simulink model "PLL_Simulering"  (R2020a)
settings: Solver=VariableStepAuto  StartTime=0  StopTime=0.5  RelTol=1e-3
InitFcn:
  | clear all;
libraries: powerlib x48, eePowerMeasurement x1, powerlib_meascontrol x1
(part 2 of 3)

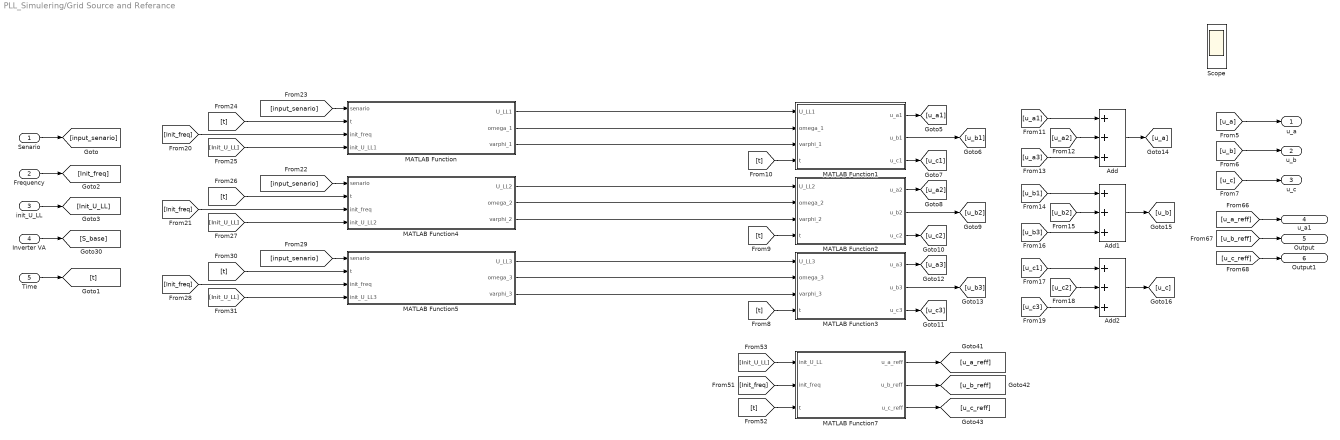
== system PLL_Simulering/Grid Source and Referance ==
  Senario : Inport
  Frequency : Inport  Port=2
  init_U_LL : Inport  Port=3
  Inverter VA : Inport  Port=4
  Time : Inport  Port=5
  Add : Sum  Inputs=+++
  Add1 : Sum  Inputs=+++
  Add2 : Sum  Inputs=+++
  MATLAB Function : MATLAB Function  TreatAsAtomicUnit=on
  MATLAB Function1 : MATLAB Function  TreatAsAtomicUnit=on
  MATLAB Function2 : MATLAB Function  TreatAsAtomicUnit=on
  MATLAB Function3 : MATLAB Function  TreatAsAtomicUnit=on
  MATLAB Function4 : MATLAB Function  TreatAsAtomicUnit=on
  MATLAB Function5 : MATLAB Function  TreatAsAtomicUnit=on
  MATLAB Function7 : MATLAB Function  TreatAsAtomicUnit=on
  Scope : Scope
  u_a : Outport
  u_b : Outport  Port=2
  u_c : Outport  Port=3
  u_a1 : Outport  Port=4
  Output : Outport  Port=5
  Output1 : Outport  Port=6
  wires:
  Senario/1 -> [input_senario]
  [u_a] -> u_a/1
  [u_c] -> u_c/1
  [u_b] -> u_b/1
  Frequency/1 -> [Init_freq]
  [t] -> MATLAB Function3/4(t)
  [t] -> MATLAB Function2/4(t)
  [t] -> MATLAB Function1/4(t)
  MATLAB Function/1(U_LL1) -> MATLAB Function1/1(U_LL1)
  MATLAB Function/2(omega_1) -> MATLAB Function1/2(omega_1)
  MATLAB Function/3(varphi_1) -> MATLAB Function1/3(varphi_1)
  init_U_LL/1 -> [Init_U_LL]
  MATLAB Function4/1(U_LL2) -> MATLAB Function2/1(U_LL2)
  MATLAB Function4/2(omega_2) -> MATLAB Function2/2(omega_2)
  MATLAB Function4/3(varphi_2) -> MATLAB Function2/3(varphi_2)
  MATLAB Function1/1(u_a1) -> [u_a1]
  MATLAB Function1/2(u_b1) -> [u_b1]
  MATLAB Function1/3(u_c1) -> [u_c1]
  MATLAB Function2/3(u_c2) -> [u_c2]
  MATLAB Function2/2(u_b2) -> [u_b2]
  MATLAB Function2/1(u_a2) -> [u_a2]
  MATLAB Function3/2(u_b3) -> [u_b3]
  MATLAB Function3/1(u_a3) -> [u_a3]
  MATLAB Function3/3(u_c3) -> [u_c3]
  [u_a1] -> Add/1
  [u_a2] -> Add/2
  [u_a3] -> Add/3
  [u_b2] -> Add1/2
  [u_b3] -> Add1/3
  [u_b1] -> Add1/1
  [u_c3] -> Add2/3
  [u_c1] -> Add2/1
  [u_c2] -> Add2/2
  Add/1 -> [u_a]
  Add1/1 -> [u_b]
  Add2/1 -> [u_c]
  [input_senario] -> MATLAB Function/1(senario)
  [t] -> MATLAB Function/2(t)
  [Init_U_LL] -> MATLAB Function/4(init_U_LL1)
  [Init_freq] -> MATLAB Function/3(init_freq)
  [Init_freq] -> MATLAB Function4/3(init_freq)
  [Init_U_LL] -> MATLAB Function4/4(init_U_LL2)
  [input_senario] -> MATLAB Function4/1(senario)
  [t] -> MATLAB Function4/2(t)
  [Init_U_LL] -> MATLAB Function5/4(init_U_LL3)
  [input_senario] -> MATLAB Function5/1(senario)
  [t] -> MATLAB Function5/2(t)
  [Init_freq] -> MATLAB Function5/3(init_freq)
  MATLAB Function5/3(varphi_3) -> MATLAB Function3/3(varphi_3)
  MATLAB Function5/2(omega_3) -> MATLAB Function3/2(omega_3)
  MATLAB Function5/1(U_LL3) -> MATLAB Function3/1(U_LL3)
  [t] -> MATLAB Function7/3(t)
  [Init_U_LL] -> MATLAB Function7/1(init_U_LL)
  [Init_freq] -> MATLAB Function7/2(init_freq)
  Inverter VA/1 -> [S_base]
  [u_a_reff] -> u_a1/1
  MATLAB Function7/1(u_a_reff) -> [u_a_reff]
  MATLAB Function7/2(u_b_reff) -> [u_b_reff]
  MATLAB Function7/3(u_c_reff) -> [u_c_reff]
  [u_b_reff] -> Output/1
  [u_c_reff] -> Output1/1
  Time/1 -> [t]

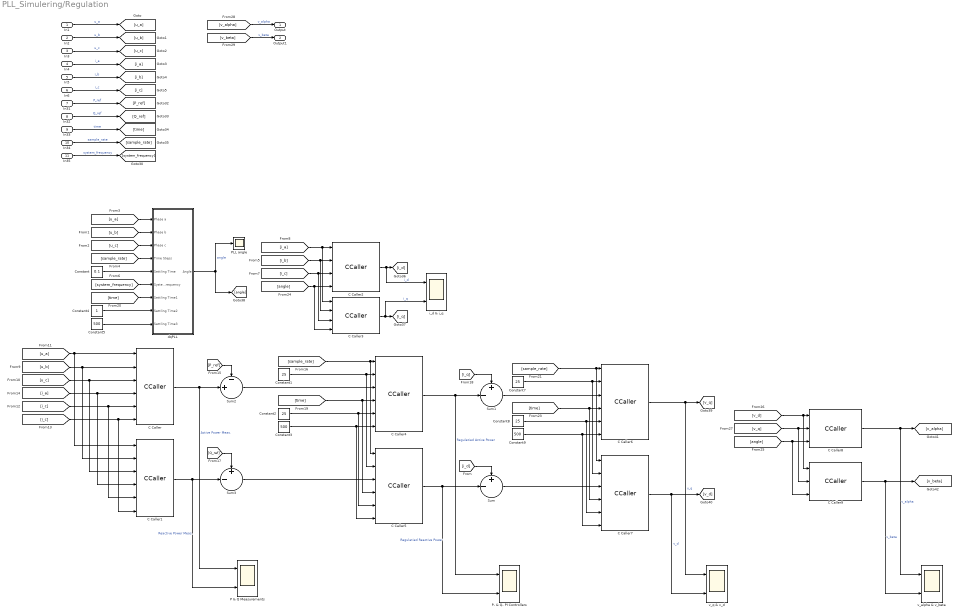
== system PLL_Simulering/Regulation ==
  In1 : Inport
  In2 : Inport  Port=2
  In3 : Inport  Port=3
  In4 : Inport  Port=4
  In5 : Inport  Port=5
  In6 : Inport  Port=6
  In31 : Inport  Port=7
  In32 : Inport  Port=8
  In33 : Inport  Port=9
  In34 : Inport  Port=10
  In35 : Inport  Port=11
  C Caller : CCaller  FunctionName=measure_P  PortSpecificationStruct="%)30     .    V L   8    (     @         %    \"     <    !     0         %  0 \"0    $    _    07)G3F%M90  4&]R=$YA;64 4V-O<&4     26YD97@     5'EP90      4VEZ90      27-';&]B86P   X    P    !@    @    $          4    (     0    ,    !         !   P!O=70 #@   #     &    \"     0         !0    @    !     P    $         $  # &]U=  .    .     8    (    !          %    \"     $    &     0         0   ...(+3703 chars)"
  C Caller1 : CCaller  FunctionName=measure_Q  PortSpecificationStruct="%)30     .    V L   8    (     @         %    \"     <    !     0         %  0 \"0    $    _    07)G3F%M90  4&]R=$YA;64 4V-O<&4     26YD97@     5'EP90      4VEZ90      27-';&]B86P   X    P    !@    @    $          4    (     0    ,    !         !   P!O=70 #@   #     &    \"     0         !0    @    !     P    $         $  # &]U=  .    .     8    (    !          %    \"     $    &     0         0   ...(+3703 chars)"
  C Caller2 : CCaller  FunctionName=Clarke_Park_d  PortSpecificationStruct="%)30     .    J @   8    (     @         %    \"     4    !     0         %  0 \"0    $    _    07)G3F%M90  4&]R=$YA;64 4V-O<&4     26YD97@     5'EP90      4VEZ90      27-';&]B86P   X    P    !@    @    $          4    (     0    ,    !         !   P!O=70 #@   #     &    \"     0         !0    @    !     P    $         $  # &]U=  .    .     8    (    !          %    \"     $    &     0         0   ...(+2601 chars)"
  C Caller3 : CCaller  FunctionName=Clarke_Park_q  PortSpecificationStruct="%)30     .    J @   8    (     @         %    \"     4    !     0         %  0 \"0    $    _    07)G3F%M90  4&]R=$YA;64 4V-O<&4     26YD97@     5'EP90      4VEZ90      27-';&]B86P   X    P    !@    @    $          4    (     0    ,    !         !   P!O=70 #@   #     &    \"     0         !0    @    !     P    $         $  # &]U=  .    .     8    (    !          %    \"     $    &     0         0   ...(+2601 chars)"
  C Caller4 : CCaller  FunctionName=PID_Type_1_1  PortSpecificationStruct="%)30     .    * P   8    (     @         %    \"     <    !     0         %  0 \"0    $    _    07)G3F%M90  4&]R=$YA;64 4V-O<&4     26YD97@     5'EP90      4VEZ90      27-';&]B86P   X    P    !@    @    $          4    (     0    ,    !         !   P!O=70 #@   #     &    \"     0         !0    @    !     P    $         $  # &]U=  .    .     8    (    !          %    \"     $    &     0         0   ...(+3810 chars)"
  C Caller5 : CCaller  FunctionName=PID_Type_1_2  PortSpecificationStruct="%)30     .    * P   8    (     @         %    \"     <    !     0         %  0 \"0    $    _    07)G3F%M90  4&]R=$YA;64 4V-O<&4     26YD97@     5'EP90      4VEZ90      27-';&]B86P   X    P    !@    @    $          4    (     0    ,    !         !   P!O=70 #@   #     &    \"     0         !0    @    !     P    $         $  # &]U=  .    .     8    (    !          %    \"     $    &     0         0   ...(+3810 chars)"
  C Caller6 : CCaller  FunctionName=PID_Type_1_3  PortSpecificationStruct="%)30     .    * P   8    (     @         %    \"     <    !     0         %  0 \"0    $    _    07)G3F%M90  4&]R=$YA;64 4V-O<&4     26YD97@     5'EP90      4VEZ90      27-';&]B86P   X    P    !@    @    $          4    (     0    ,    !         !   P!O=70 #@   #     &    \"     0         !0    @    !     P    $         $  # &]U=  .    .     8    (    !          %    \"     $    &     0         0   ...(+3810 chars)"
  C Caller7 : CCaller  FunctionName=PID_Type_1_4  PortSpecificationStruct="%)30     .    * P   8    (     @         %    \"     <    !     0         %  0 \"0    $    _    07)G3F%M90  4&]R=$YA;64 4V-O<&4     26YD97@     5'EP90      4VEZ90      27-';&]B86P   X    P    !@    @    $          4    (     0    ,    !         !   P!O=70 #@   #     &    \"     0         !0    @    !     P    $         $  # &]U=  .    .     8    (    !          %    \"     $    &     0         0   ...(+3810 chars)"
  C Caller8 : CCaller  FunctionName=Park_inv_alpha  PortSpecificationStruct="%)30     .    \" <   8    (     @         %    \"     0    !     0         %  0 \"0    $    _    07)G3F%M90  4&]R=$YA;64 4V-O<&4     26YD97@     5'EP90      4VEZ90      27-';&]B86P   X    P    !@    @    $          4    (     0    ,    !         !   P!O=70 #@   #     &    \"     0         !0    @    !     P    $         $  # &]U=  .    .     8    (    !          %    \"     $    &     0         0  ...(+2044 chars)"
  C Caller9 : CCaller  FunctionName=Park_inv_beta  PortSpecificationStruct="%)30     .    \" <   8    (     @         %    \"     0    !     0         %  0 \"0    $    _    07)G3F%M90  4&]R=$YA;64 4V-O<&4     26YD97@     5'EP90      4VEZ90      27-';&]B86P   X    P    !@    @    $          4    (     0    ,    !         !   P!O=70 #@   #     &    \"     0         !0    @    !     P    $         $  # &]U=  .    .     8    (    !          %    \"     $    &     0         0  ...(+2044 chars)"
  Constant : Constant  Value=0.1
  Constant{1..2,7..8} (4 alike) : Constant  Value=25
  Constant3 : Constant  Value=500
  Constant4 : Constant
  Constant5 : Constant  Value=500
  Constant9 : Constant  Value=500
  P & Q Measurements : Scope  NumInputPorts=2
  P- & Q- PI Controllers : Scope  NumInputPorts=2
  PLL angle : Scope
  Sum : Sum  Inputs=+-|
  Sum1 : Sum  Inputs=+-|
  Sum2 : Sum  Inputs=-+|
  Sum3 : Sum  Inputs=+-|
  dqPLL : Subsystem
  i_d & i_q : Scope  NumInputPorts=2
  v_alpha & v_beta : Scope  NumInputPorts=2
  v_q & v_d : Scope  NumInputPorts=2
  Output : Outport
  Output1 : Outport  Port=2
  wires:
  In1/1 -> [u_a]  "u_a"
  In2/1 -> [u_b]  "u_b"
  In3/1 -> [u_c]  "u_c"
  In4/1 -> [i_a]  "i_a"
  In5/1 -> [i_b]  "i_b"
  In6/1 -> [i_c]  "i_c"
  In33/1 -> [time]  "time"
  In31/1 -> [P_ref]  "P_ref"
  In35/1 -> [system_frequency]  "system_frequency"
  In34/1 -> [sample_rate]  "sample_rate"
  In32/1 -> [Q_ref]  "Q_ref"
  [u_a] -> dqPLL/1(Phase a)
  [u_b] -> dqPLL/2(Phase b)
  [u_c] -> dqPLL/3(Phase c)
  Constant/1 -> dqPLL/5(Settling Time)
  [system_frequency] -> dqPLL/6(System Frequency)
  [sample_rate] -> dqPLL/4(Time Steps)
  [i_a] -> C Caller3/1, C Caller2/1
  [i_b] -> C Caller3/2, C Caller2/2
  [i_c] -> C Caller3/3, C Caller2/3
  [u_a] -> C Caller1/1, C Caller/1
  [u_b] -> C Caller1/2, C Caller/2
  [u_c] -> C Caller/3, C Caller1/3
  [i_a] -> C Caller1/4, C Caller/4
  [i_c] -> C Caller/5, C Caller1/5
  [i_c] -> C Caller1/6, C Caller/6
  [sample_rate] -> C Caller5/1, C Caller4/1
  Constant1/1 -> C Caller5/2, C Caller4/2
  C Caller/1 -> Sum2/2, P & Q Measurements/1  "Active Power Meas."
  [time] -> C Caller5/4, C Caller4/4
  Constant2/1 -> C Caller5/5, C Caller4/5
  Constant3/1 -> C Caller5/6, C Caller4/6
  C Caller1/1 -> Sum3/2, P & Q Measurements/2  "Reactive Power Meas."
  C Caller5/1 -> P- & Q- PI Controllers/2, Sum/2  "Regulatied Reactive Power"
  C Caller2/1 -> i_d & i_q/1, [i_d]  "i_d"
  C Caller3/1 -> i_d & i_q/2, [i_q]  "i_q"
  [i_d] -> Sum/1
  [i_q] -> Sum1/1
  C Caller4/1 -> P- & Q- PI Controllers/1, Sum1/2  "Regulatied Active Power"
  [sample_rate] -> C Caller7/1, C Caller6/1
  Sum1/1 -> C Caller6/3
  Constant8/1 -> C Caller7/5, C Caller6/5
  Constant9/1 -> C Caller7/6, C Caller6/6
  [time] -> C Caller7/4, C Caller6/4
  Sum/1 -> C Caller7/3
  Constant7/1 -> C Caller7/2, C Caller6/2
  dqPLL/1(Angle) -> [angle], PLL angle/1  "angle"
  [angle] -> C Caller3/4, C Caller2/4
  C Caller6/1 -> v_q & v_d/1, [v_q]  "v_q"
  C Caller7/1 -> v_q & v_d/2, [v_d]  "v_d"
  [v_d] -> C Caller9/1, C Caller8/1
  [v_q] -> C Caller9/2, C Caller8/2
  [angle] -> C Caller9/3, C Caller8/3
  C Caller8/1 -> v_alpha & v_beta/1, [v_alpha]  "v_alpha"
  C Caller9/1 -> v_alpha & v_beta/2, [v_beta]  "v_beta"
  [v_alpha] -> Output/1  "v_alpha"
  [v_beta] -> Output1/1  "v_beta"
  Sum2/1 -> C Caller4/3
  [P_ref] -> Sum2/1
  [Q_ref] -> Sum3/1
  Sum3/1 -> C Caller5/3
  [time] -> dqPLL/7(Settling Time1)
  Constant4/1 -> dqPLL/8(Settling Time2)
  Constant5/1 -> dqPLL/9(Settling Time3)
